simulink model "observer"  (R2017a)
settings: Solver=VariableStepAuto  StartTime=0.0  StopTime=10.0  RelTol=1e-3
values from neighbouring files (symbols this model uses):
  A = [0 a12   0   0 ... (first row only)    [Lab6b.m]    (also in prelab6b.m)
  C = [1 0 0 0 ... (first row only)    [Lab6b.m]    (also in prelab6b.m = [1 0 0 0; 0 0 1 0])
  ref = [0 0 0 0]    [Lab6b.m]
undefined symbols (not defined in the file or in its folder): A_k, B_k
settings Model: Creator=trey  LastModifiedBy=trey

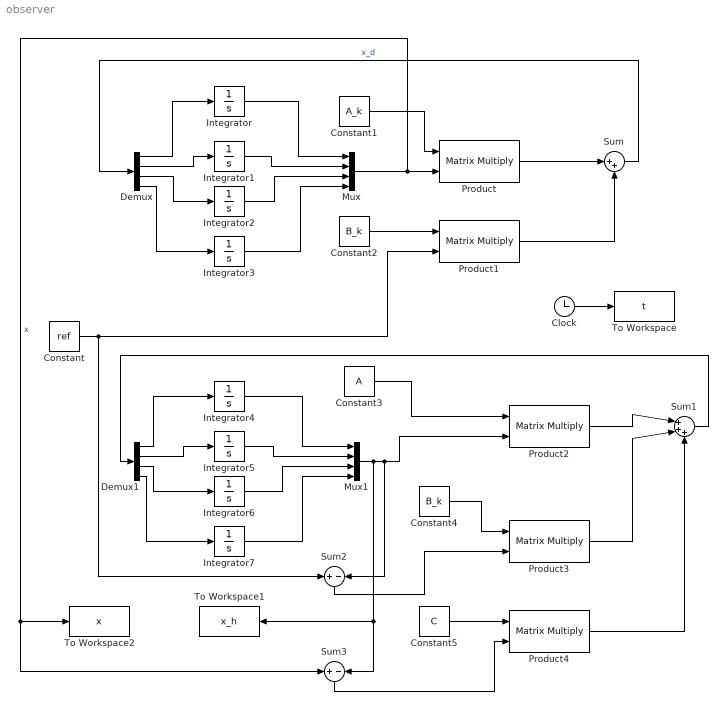
== system observer ==
  Clock : Clock
  Constant : Constant  Value=ref
  Constant1 : Constant  Value=A_k
  Constant2 : Constant  Value=B_k
  Constant3 : Constant  Value=A
  Constant4 : Constant  Value=B_k
  Constant5 : Constant  Value=C
  Demux : Demux
  Demux1 : Demux
  Integrator{,1..7} (8 alike) : Integrator
  Mux : Mux
  Mux1 : Mux
  Product{,1..4} (5 alike) : Product  Multiplication=Matrix(*)
  Sum : Sum  Inputs=|++
  Sum1 : Sum  Inputs=|+++
  Sum2 : Sum  Inputs=+-
  Sum3 : Sum  Inputs=+-
  To Workspace : ToWorkspace  VariableName=t  SaveFormat=Timeseries  SampleTime=-1
  To Workspace1 : ToWorkspace  VariableName=x_h  SaveFormat=Timeseries  SampleTime=-1
  To Workspace2 : ToWorkspace  VariableName=x  SaveFormat=Timeseries  SampleTime=-1
  wires:
  Demux/1 -> Integrator/1
  Demux/2 -> Integrator1/1
  Demux/3 -> Integrator2/1
  Demux/4 -> Integrator3/1
  Integrator/1 -> Mux/1
  Integrator1/1 -> Mux/2
  Integrator2/1 -> Mux/3
  Integrator3/1 -> Mux/4
  Mux/1 -> Sum3/1, To Workspace2/1, Product/2  "x"
  Product/1 -> Sum/1
  Sum/1 -> Demux/1  "x_d"
  Constant/1 -> Sum2/1, Product1/2
  Constant1/1 -> Product/1
  Constant2/1 -> Product1/1
  Product1/1 -> Sum/2
  Demux1/1 -> Integrator4/1
  Demux1/2 -> Integrator5/1
  Demux1/3 -> Integrator6/1
  Demux1/4 -> Integrator7/1
  Integrator4/1 -> Mux1/1
  Integrator5/1 -> Mux1/2
  Integrator6/1 -> Mux1/3
  Integrator7/1 -> Mux1/4
  Mux1/1 -> Sum3/2, To Workspace1/1, Sum2/2, Product2/2
  Constant3/1 -> Product2/1
  Product2/1 -> Sum1/1
  Constant4/1 -> Product3/1
  Constant5/1 -> Product4/1
  Clock/1 -> To Workspace/1
  Product3/1 -> Sum1/2
  Product4/1 -> Sum1/3
  Sum1/1 -> Demux1/1
  Sum2/1 -> Product3/2
  Sum3/1 -> Product4/2
